simulink model "ej7"  (R2023a)
settings: Solver=VariableStepAuto  StartTime=0.0  StopTime=30  MaxStep=1e-4  RelTol=1e-3
settings Model: Creator=Juan  LastModifiedBy=Juan

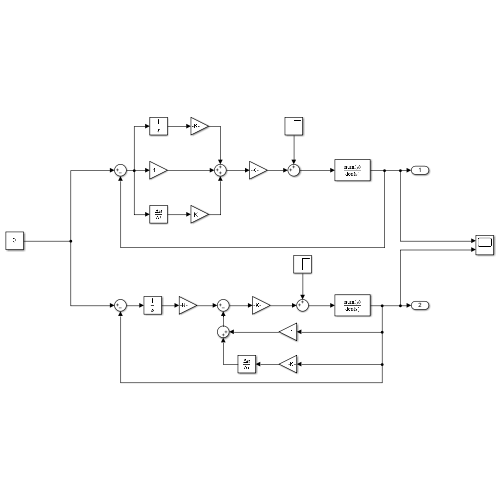
[thumbnail: Simulink's stored preview of the top-level diagram]
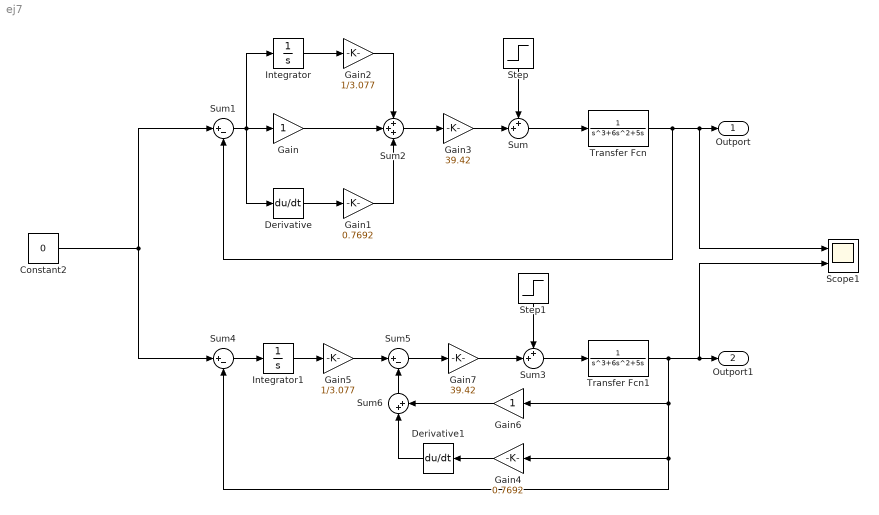
== system ej7 ==
  Constant2 : Constant  Value=0
  Derivative : Derivative
  Derivative1 : Derivative
  Gain : Gain
  Gain1 : Gain  Gain=0.7692
  Gain2 : Gain  Gain=1/3.077
  Gain3 : Gain  Gain=39.42
  Gain4 : Gain  Gain=0.7692
  Gain5 : Gain  Gain=1/3.077
  Gain6 : Gain
  Gain7 : Gain  Gain=39.42
  Integrator : Integrator
  Integrator1 : Integrator
  Scope1 : Scope  NumInputPorts=2
  Step : Step  Time=2  After=10  SampleTime=0
  Step1 : Step  Time=2  After=10  SampleTime=0
  Sum : Sum  Inputs=++|
  Sum1 : Sum  Inputs=|+-
  Sum2 : Sum  Inputs=+++
  Sum3 : Sum  Inputs=++|
  Sum4 : Sum  Inputs=|+-
  Sum5 : Sum  Inputs=|+-
  Sum6 : Sum  Inputs=|++
  Transfer Fcn : TransferFcn  Denominator=[1 6 5 0]
  Transfer Fcn1 : TransferFcn  Denominator=[1 6 5 0]
  Outport : Outport
  Outport1 : Outport  Port=2
  wires:
  Sum/1 -> Transfer Fcn/1
  Sum1/1 -> Derivative/1, Integrator/1, Gain/1
  Transfer Fcn/1 -> Sum1/2, Scope1/1, Outport/1
  Gain/1 -> Sum2/2
  Derivative/1 -> Gain1/1
  Integrator/1 -> Gain2/1
  Gain2/1 -> Sum2/1
  Gain1/1 -> Sum2/3
  Sum2/1 -> Gain3/1
  Step/1 -> Sum/1
  Sum5/1 -> Gain7/1
  Constant2/1 -> Sum1/1, Sum4/1
  Step1/1 -> Sum3/1
  Sum3/1 -> Transfer Fcn1/1
  Transfer Fcn1/1 -> Gain6/1, Gain4/1, Sum4/2, Scope1/2, Outport1/1
  Gain5/1 -> Sum5/1
  Integrator1/1 -> Gain5/1
  Sum4/1 -> Integrator1/1
  Gain3/1 -> Sum/2
  Gain4/1 -> Derivative1/1
  Derivative1/1 -> Sum6/1
  Gain6/1 -> Sum6/2
  Sum6/1 -> Sum5/2
  Gain7/1 -> Sum3/2
